simulink model "DynamicsAndKinematics"  (Simulink 8.5)
settings: Solver=ode1  StartTime=0.0  StopTime=20000  FixedStep=0.1  RelTol=1e-3
InitFcn:
  | % Bifocal Relay Mirror Spacecraft (prior to payload installation) Dynamics Simulation      TA Sands
  | clear all;close all;clc;warning off all;
  | 
  | % Simulation run parameters
  | Rate=34.3; DeltaT=1/Rate;
  | 
  | % Maneuver Parameters
  | roll=0; pitch=0; yaw=30; roll=roll*pi/180; pitch=pitch*pi/180; yaw=yaw*pi/180;
  | SlewTime=5; SACengage=0;
  | 
  | %Constants0
  | Re=6371.2e3;mu=398601.2e9; %earth radius and universal gravitation constant
  | 
  | %Spacecraft orbit
  | h=180e3; %orbit altitude in meters
  | R=Re+h; %orbit radius from center of earth
  | we=0.000072921158553; %earth's angular velocity rad/solar sec(Vallado)
  | wo=sqrt(mu/(Re+h)^3); %orbit angular velocity
  | incln=36.6001*pi/180; %Inclination assumed Monterey Latitude
  | epsilon=12*pi/180; alphao=0;
  | uo=0; nuo=0; %Start S/C beneath subsolar point
  | beta=60; gamma=1.5;
  | a=0.545491852; b=0.314939867; c=0.704226952; %Assumed spacecraft rectangular size
  | Area=[b*c a*c a*b]; %projected area~m^2 in body x,y,z directions
  | density=4.39e-14;
  | kpre=-9.9639/24/3600/180*pi*0; %nodal precession constant assumed zero here
  | wn=kpre*(Re/(Re+h))^3.5*cos(incln); %nodal precession (zero eccentricity)
  | V=wo*(Re+h);
  | rho=asin(Re/(h+Re)); %earth angular radius
  | Cd=2.5; psun=4.5E-6; %Drag coefficient and solar pressure constant~N/m^2
  | Kaero=-0.5*Cd*V^2; Psolar=2*psun; %constants for aero and solar torque calculation
  | dL=[0.002 0.002 0.008]; %predicted distance between cp and cg
  | Kme=2.3390e-005;
  | 
  | %Spacecraft Magnetic Properties (assumed)
  | mresid=[0 0 0.01]; %Spacecraft residual magnetic moment
  | M=mresid; %Magnetic unit dipole vector
  | K=7.943e15;
  | 
  | %Spacecraft Inertia conditions
  | Ix=119.1259; Iy=150.6615; Iz=106.0288;
  | Ixy=-15.76781; Iyz=22.3164; Ixz=-6.5486;
  | Imo=[Ix Ixy Ixz;
  | Ixy Iy Iyz;
  | Ixz Iyz Iz]; %Moment of inertia matrix
  | Iinv=inv(Imo); %Moment of inertia inverse goes in dynamics block
  | 
  |  %Decoupled Inertia
  | Imo2=[119.1259 0 0;
  | 0 150.6615 0;
  | 0 0 106.0288];
  | Iinv2=inv(Imo2);
  | 
  | %Spacecraft initial Euler state angles and rates
  | phio=0;thetao=0;psio=0; %Initial Euler Angles
  | phidoto=0;thetadoto=0;psidoto=0; %Initial Euler Rates
  | 
  | %Calculation of initial quaternion (qo) and angular momentum (Ho)
  | s1=sin(phio/2);s2=sin(thetao/2);s3=sin(psio/2);c1=cos(phio/2);c2=cos(thetao/2);c3=cos(psio/2);
  | q1o=s1*c2*c3-c1*s2*s3;
  | q2o=c1*s2*c3+s1*c2*s3; %Wie pg. 321
  | q3o=c1*c2*s3-s1*s2*c3;
  | q4o=c1*c2*c3+s1*s2*s3;
  | S1=sin(phio);S2=sin(thetao);S3=sin(psio);C1=cos(phio);C2=cos(thetao);C3=cos(psio);
  | wxo=phidoto-psidoto*S2-wo*S3*C2;
  | wyo=thetadoto*C1+psidoto*C2*S1-wo*(C3*C1+S3*S2*S1);
  | wzo=psidoto*C2*C1-thetadoto*S1-wo*(S3*S2*C1-C3*S1);
  | qo=[q1o q2o q3o q4o];
  | Ho=Imo*[wxo wyo wzo]';
  | norm(Ho)*1000;
  | 
  | %Calculate eclipse time for comparison with EPS calculations
  | Te=100.87*2*V/2/pi;
  | 
  | 
  | 
StopFcn:
  | h2=figure;
  | plot(clock,Euler),title('Full Simulation Euler Angles'),xlabel('time(sec)'),ylabel('Angles (degrees)'),grid
  | 
  | 
  | figure(6);
  | 
  | EulerX=Euler(:,1);EulerY=Euler(:,2);EulerZ=Euler(:,3);
  | 
  | 
  | 
  | subplot(3,1,1);plot(clock,EulerX,'linewidth',2); axis([0,20000,min(EulerX)*5,max(EulerX)*5]);grid;ylabel('\phi(deg)','fontsize',10);title('Error Euler Angles','fontsize',14); set(gca,'XTickLabel',{' ',' ',' ',' ',' ',' ',' ',' ','10'}); set(gca,'fontsize',10);
  | subplot(3,1,2);plot(clock,EulerY,'linewidth',2); axis([0,20000,min(EulerY)*5,max(EulerY)*5]); grid;ylabel('\theta(deg)','fontsize',10); set(gca,'XTickLabel',{' ',' ',' ',' ',' ',' ',' ',' ','10'}); set(gca,'fontsize',10);
  | subplot(3,1,3);plot(clock,EulerZ,'linewidth',2);axis([0,20000,min(EulerZ)*1.25,max(EulerZ)*1.25]);grid; ylabel('\psi(deg)','fontsize',10); set(gca,'XTickLabel',{' ',' ',' ',' ',' ',' ',' ',' ','10'}); set(gca,'fontsize',10);
  | 
  | %STDx=std(ERROR(:,1));
  | 
  | %STDy=std(ERROR(:,2));
  | 
  | %STDz=std(ERROR(:,3));
  | 
  | 
  | %subplot(4,1,4);plot(clock,STDx,'blue','linewidth',2);axis([0,20000,min(EulerZ)*1.25,max(EulerZ)*1.25]);grid;
  | %hold on
  | %subplot(4,1,4);plot(clock,STDy,'blue','linewidth',2);axis([0,20000,min(EulerZ)*1.25,max(EulerZ)*1.25]);grid;
  | %subplot(4,1,4);plot(clock,STDz,'black','linewidth',2);axis([0,20000,min(EulerZ)*1.25,max(EulerZ)*1.25]);grid;
  | %ylabel('\psi(deg)','fontsize',10); set(gca,'XTickLabel',{' ',' ',' ',' ',' ',' ',' ',' ','10'}); set(gca,'fontsize',10);
  | %xlabel('Time(s)'),ylabel('Euler Error (degrees)'),grid
  | %hold off
libraries: simulink x1, aerospace x1
settings Model: Creator=grompone  LastModifiedBy=Acer
settings OptimizationCC: InitFltsAndDblsToZero=on
settings DebuggingCC: SaveWithParameterizedLinksMsg=none  SolverPrmCheckMsg=warning  FcnCallInpInsideContextMsg=UseLocalSettings  StrictBusMsg=Warning
settings SFSimCC: SimParseCustomCode=off
settings GRTTargetCC: TargetFcnLib=ansi_tfl_tmw.mat

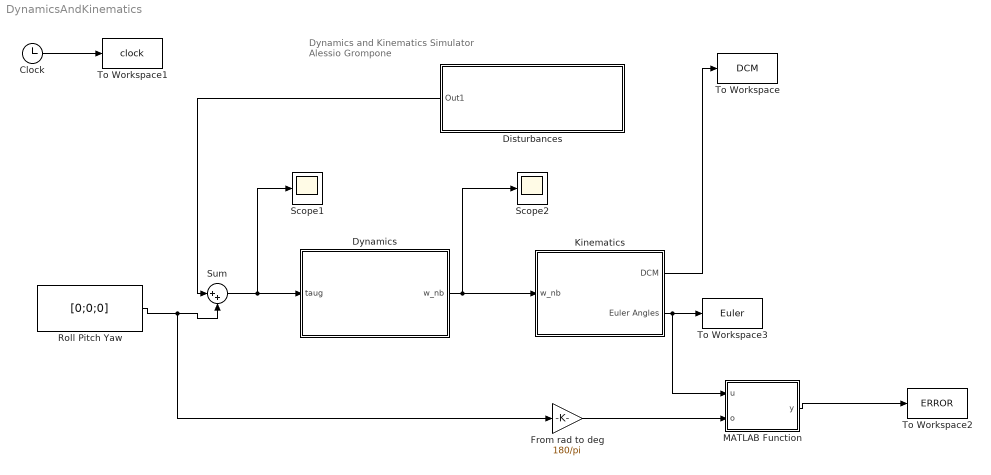
== system DynamicsAndKinematics ==
  note: Dynamics and Kinematics Simulator
      | Alessio Grompone
  Clock : Clock
  Disturbances : Subsystem
  Dynamics : Subsystem
  From rad to deg : Gain  Gain=180/pi
  Kinematics : Subsystem
  MATLAB Function : MATLAB Function  TreatAsAtomicUnit=on
  Roll Pitch Yaw : Constant  Value=[0;0;0]
  Scope1 : Scope
      settings: SaveName=ScopeData2
  Scope2 : Scope
  Sum : Sum  Inputs=|++
  To Workspace : ToWorkspace  VariableName=DCM  SampleTime=-1
  To Workspace1 : ToWorkspace  VariableName=clock  SampleTime=-1
  To Workspace2 : ToWorkspace  VariableName=ERROR  SampleTime=-1
  To Workspace3 : ToWorkspace  VariableName=Euler  SampleTime=-1
  wires:
  Dynamics/1(w_nb) -> Scope2/1, Kinematics/1(w_nb)
  Clock/1 -> To Workspace1/1
  Kinematics/1(DCM) -> To Workspace/1
  Roll Pitch Yaw/1 -> Sum/2, From rad to deg/1
  Disturbances/1(Out1) -> Sum/1
  Sum/1 -> Dynamics/1(taug), Scope1/1
  Kinematics/2(Euler Angles) -> To Workspace3/1, MATLAB Function/1(u)
  MATLAB Function/1(y) -> To Workspace2/1
  From rad to deg/1 -> MATLAB Function/2(o)

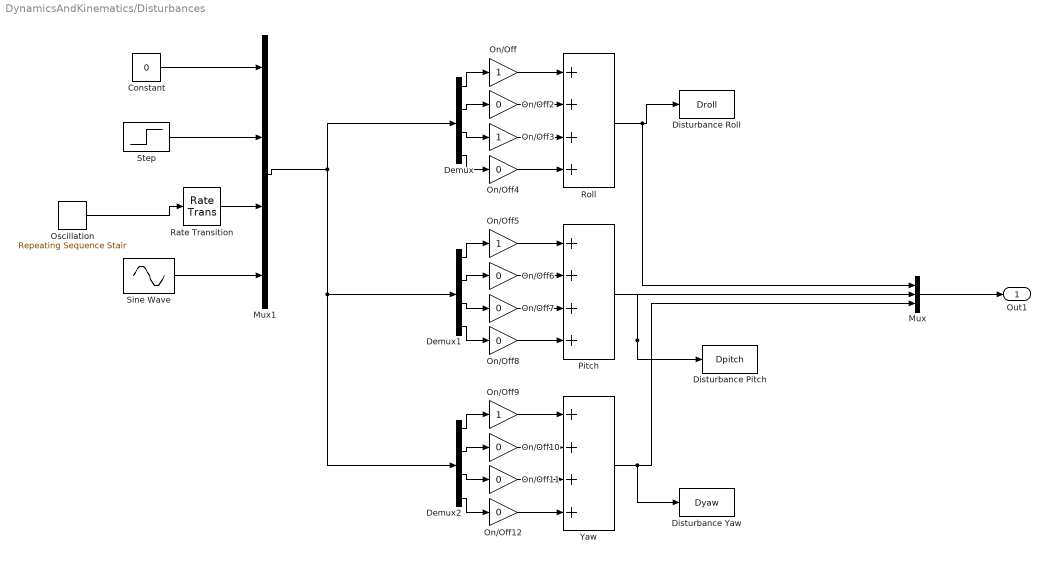
== system DynamicsAndKinematics/Disturbances ==
  Constant : Constant  Value=0
  Demux : Demux
  Demux1 : Demux
  Demux2 : Demux
  Disturbance Pitch : ToWorkspace  VariableName=Dpitch  SampleTime=-1
  Disturbance Roll : ToWorkspace  VariableName=Droll  SampleTime=-1
  Disturbance Yaw : ToWorkspace  VariableName=Dyaw  SampleTime=-1
  Mux : Mux  Inputs=3
  Mux1 : Mux
  On/Off{,3,5,9} (4 alike) : Gain  SaturateOnIntegerOverflow=on  OutDataTypeStr=Inherit: Same as input  ParamDataTypeStr=Inherit: Same as input
  On/Off{2,4,6..8,10..12} (8 alike) : Gain  Gain=0  SaturateOnIntegerOverflow=on  OutDataTypeStr=Inherit: Same as input  ParamDataTypeStr=Inherit: Same as input
  Oscillation : simulink/Sources/Repeating Sequence Stair  OutValues=[ 0.01 -0.01 -0.01 0.01]  tsamp=10  OutMin=[]  OutMax=[]  OutDataTypeStr=double  OutputDataTypeScalingMode=double  OutDataType=fixdt(0,8)  ConRadixGroup=Best Precision: Vector-wise  OutScaling=2^-12
  Pitch : Sum  Inputs=++++
  Rate Transition : RateTransition
  Roll : Sum  Inputs=++++
  Sine Wave : Sin  Amplitude=.1  Frequency=0.1  SampleTime=0  VectorParams1D=off
  Step : Step  Time=40  After=0.1  SampleTime=0
  Yaw : Sum  Inputs=++++
  Out1 : Outport
  wires:
  On/Off/1 -> Roll/1
  On/Off2/1 -> Roll/2
  On/Off3/1 -> Roll/3
  On/Off4/1 -> Roll/4
  On/Off5/1 -> Pitch/1
  On/Off6/1 -> Pitch/2
  On/Off7/1 -> Pitch/3
  On/Off8/1 -> Pitch/4
  On/Off9/1 -> Yaw/1
  On/Off10/1 -> Yaw/2
  On/Off11/1 -> Yaw/3
  On/Off12/1 -> Yaw/4
  Roll/1 -> Disturbance Roll/1, Mux/1
  Pitch/1 -> Disturbance Pitch/1, Mux/2
  Yaw/1 -> Disturbance Yaw/1, Mux/3
  Demux/1 -> On/Off/1
  Demux/2 -> On/Off2/1
  Demux/3 -> On/Off3/1
  Demux/4 -> On/Off4/1
  Demux1/1 -> On/Off5/1
  Demux1/2 -> On/Off6/1
  Demux1/3 -> On/Off7/1
  Demux1/4 -> On/Off8/1
  Demux2/1 -> On/Off9/1
  Demux2/2 -> On/Off10/1
  Demux2/3 -> On/Off11/1
  Demux2/4 -> On/Off12/1
  Constant/1 -> Mux1/1
  Step/1 -> Mux1/2
  Mux/1 -> Out1/1
  Mux1/1 -> Demux/1, Demux1/1, Demux2/1
  Sine Wave/1 -> Mux1/4
  Rate Transition/1 -> Mux1/3
  Oscillation/1 -> Rate Transition/1

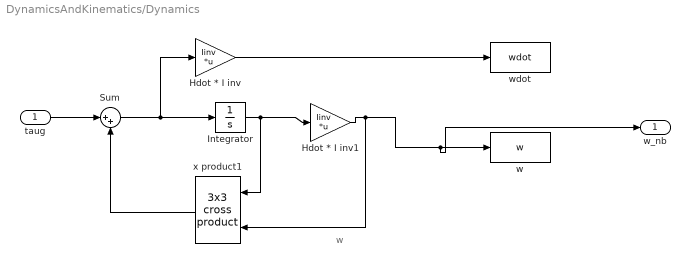
== system DynamicsAndKinematics/Dynamics ==
  note: w
  taug : Inport
  "  Hdot * I inv" : Gain  Gain=Iinv  Multiplication=Matrix(K*u)  SaturateOnIntegerOverflow=on  OutDataTypeStr=Inherit: Same as input  ParamDataTypeStr=Inherit: Same as input
  "  Hdot * I inv1" : Gain  Gain=Iinv  Multiplication=Matrix(K*u)  SaturateOnIntegerOverflow=on  OutDataTypeStr=Inherit: Same as input  ParamDataTypeStr=Inherit: Same as input
  Integrator : Integrator  InitialCondition=[0;0;0]
  Sum : Sum  Inputs=|++
  w : ToWorkspace  VariableName=w  SampleTime=-1
  wdot : ToWorkspace  VariableName=wdot  SampleTime=-1
  x product1 : aerospace/Axes Transformations/3x3 cross product
  w_nb : Outport
  wires:
  Integrator/1 -> x product1/1, "  Hdot * I inv1"/1
  taug/1 -> Sum/1
  x product1/1 -> Sum/2
  Sum/1 -> "  Hdot * I inv"/1, Integrator/1
  "  Hdot * I inv"/1 -> wdot/1
  "  Hdot * I inv1"/1 -> x product1/2, w/1, w_nb/1

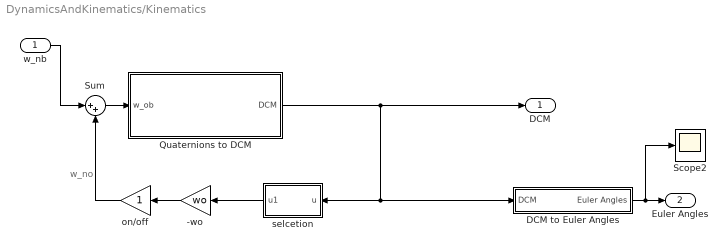
== system DynamicsAndKinematics/Kinematics ==
  note: w_no
  w_nb : Inport
  -wo : Gain  Gain=wo
  DCM to Euler Angles : Subsystem
  Quaternions to DCM : Subsystem
  Scope2 : Scope
      settings: YMin=-60  YMax=60  SaveName=ScopeData3
  Sum : Sum  Inputs=|++
  on/off : Gain
  "selcetion " : MATLAB Function  TreatAsAtomicUnit=on
  DCM : Outport
  Euler Angles : Outport  Port=2
  wires:
  w_nb/1 -> Sum/1
  Quaternions to DCM/1(DCM) -> DCM/1, "selcetion "/1(u), DCM to Euler Angles/1(DCM)
  Sum/1 -> Quaternions to DCM/1(w_ob)
  on/off/1 -> Sum/2
  "selcetion "/1(u1) -> -wo/1
  -wo/1 -> on/off/1
  DCM to Euler Angles/1(Euler Angles) -> Euler Angles/1, Scope2/1

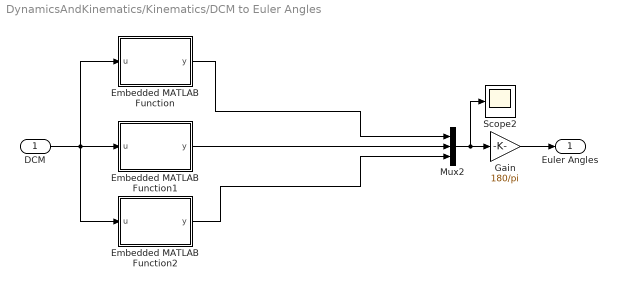
== system DynamicsAndKinematics/Kinematics/DCM to Euler Angles ==
  DCM : Inport
  Embedded MATLAB Function : MATLAB Function  TreatAsAtomicUnit=on
  Embedded MATLAB Function1 : MATLAB Function  TreatAsAtomicUnit=on
  Embedded MATLAB Function2 : MATLAB Function  TreatAsAtomicUnit=on
  Gain : Gain  Gain=180/pi
  Mux2 : Mux  Inputs=3
  Scope2 : Scope
      settings: SaveName=ScopeData7
  Euler Angles : Outport
  wires:
  Embedded MATLAB Function/1(y) -> Mux2/1
  Embedded MATLAB Function2/1(y) -> Mux2/3
  Embedded MATLAB Function1/1(y) -> Mux2/2
  DCM/1 -> Embedded MATLAB Function1/1(u), Embedded MATLAB Function/1(u), Embedded MATLAB Function2/1(u)
  Mux2/1 -> Gain/1, Scope2/1
  Gain/1 -> Euler Angles/1

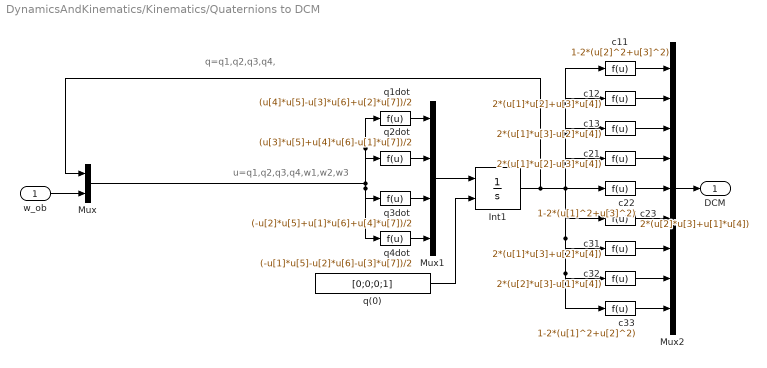
== system DynamicsAndKinematics/Kinematics/Quaternions to DCM ==
  note: q=q1,q2,q3,q4,
  note: u=q1,q2,q3,q4,w1,w2,w3
  w_ob : Inport
  Int1 : Integrator  InitialConditionSource=external  InitialCondition=[0 0 -0.1]'
  Mux : Mux  Inputs=2
  Mux1 : Mux
  Mux2 : Mux  Inputs=9
  c11 : Fcn  Expr=1-2*(u[2]^2+u[3]^2)
  c12 : Fcn  Expr=2*(u[1]*u[2]+u[3]*u[4])
  c13 : Fcn  Expr=2*(u[1]*u[3]-u[2]*u[4])
  c21 : Fcn  Expr=2*(u[1]*u[2]-u[3]*u[4])
  c22 : Fcn  Expr=1-2*(u[1]^2+u[3]^2)
  c23 : Fcn  Expr=2*(u[2]*u[3]+u[1]*u[4])
  c31 : Fcn  Expr=2*(u[1]*u[3]+u[2]*u[4])
  c32 : Fcn  Expr=2*(u[2]*u[3]-u[1]*u[4])
  c33 : Fcn  Expr=1-2*(u[1]^2+u[2]^2)
  q(0) : Constant  Value=[0;0;0;1]
  q1dot : Fcn  Expr=(u[4]*u[5]-u[3]*u[6]+u[2]*u[7])/2
  q2dot : Fcn  Expr=(u[3]*u[5]+u[4]*u[6]-u[1]*u[7])/2
  q3dot : Fcn  Expr=(-u[2]*u[5]+u[1]*u[6]+u[4]*u[7])/2
  q4dot : Fcn  Expr=(-u[1]*u[5]-u[2]*u[6]-u[3]*u[7])/2
  DCM : Outport
  wires:
  Mux/1 -> q4dot/1, q3dot/1, q1dot/1, q2dot/1
  q1dot/1 -> Mux1/1
  q2dot/1 -> Mux1/2
  q3dot/1 -> Mux1/3
  q4dot/1 -> Mux1/4
  Int1/1 -> Mux/1, c22/1, c21/1, c13/1, c12/1, c11/1, c23/1, c31/1, c32/1, c33/1
  Mux1/1 -> Int1/1
  q(0)/1 -> Int1/2
  c11/1 -> Mux2/1
  c12/1 -> Mux2/2
  c13/1 -> Mux2/3
  c21/1 -> Mux2/4
  c22/1 -> Mux2/5
  c23/1 -> Mux2/6
  c31/1 -> Mux2/7
  c32/1 -> Mux2/8
  c33/1 -> Mux2/9
  w_ob/1 -> Mux/2
  Mux2/1 -> DCM/1

== matlab function Kinematics/DCM to Euler Angles/Embedded MATLAB Function ==
  data: u input double; y output double
function y = fcn(u)
% This block supports an embeddable subset of the MATLAB language.
% See the help menu for details. 

y = u(6);

== matlab function Kinematics/selcetion  ==
  data: u input double; u1 output double
function u1  = Select(u)
% This block supports an embeddable subset of the MATLAB language.
% See the help menu for details. 

u11=u(2);

u22=u(5);

u33=u(8);

u1=[u11;u22;u33];

== matlab function Kinematics/DCM to Euler Angles/Embedded MATLAB Function1 ==
  data: u input double; y output double
function y = fcn(u)
% This block supports an embeddable subset of the MATLAB language.
% See the help menu for details. 

y = -asin(u(3));

== matlab function Kinematics/DCM to Euler Angles/Embedded MATLAB Function2 ==
  data: u input double; y output double
function y = fcn(u)
% This block supports an embeddable subset of the MATLAB language.
% See the help menu for details. 

y = u(2);

== matlab function MATLAB Function ==
  data: u input double; y output double; o input double
function y = fcn(u,o)
%#codegen
y=[0,0,0];

y(1) =u(1)-o(1);
y(2) =u(2)-o(2);
y(3) =u(3)-o(3);
